simulink model "CalebsModel_v3"  (Simulink 8.3)
settings: Solver=ode45  StartTime=0.0  StopTime=60  RelTol=1e-3
values from neighbouring files (symbols this model uses):
  a_lim = 0.75*F_max/Mar    (= 600)    [ControlDesign.m]
  b_surf = 1e5    (= 100000)    [ControlDesign.m]
  bp = 100    [ControlDesign.m]
  ContactPoint = 0.023    [ControlDesign.m]
  F_max = 60    [ControlDesign.m]
  Home = 0    [ControlDesign.m]
  k_1 = (z_1*z_2-1+k_2*Ts)/(k_2*Ts^2)    [ControlDesign.m]
  k_2 = (2-(z_1+z_2))/Ts    [ControlDesign.m]
  K_backemf = 1000*mean( K_backemf_array )    [ControlDesign.m]
  K_L12_Force = 0.00229181    [ControlDesign.m]    (also in ControlDesignForceModeLinear.m = 2.29181)
  K_PWM = PWM_res/V_rail    (= 83.3333333333)    [ControlDesign.m]    (also in ControlDesignForceModeLinear.m = 0.012)
  k_surf = 1e8    (= 100000000)    [ControlDesign.m]
  kvc = 20e3    (= 20000)    [ControlDesign.m]
  L12_Offset_I = 0.012995    [ControlDesign.m]    (also in ControlDesignForceModeLinear.m = 12.995)
  L_Range = [0 0.050]    [ControlDesign.m]    (also in ControlDesignForceModeLinear.m = [0 50]; VariableQpts.m = [0 50])
  m_surf = 1e3    (= 1000)    [ControlDesign.m]
  Mar = 0.075    [ControlDesign.m]    (also in ControlDesignForceModeLinear.m)
  PWM_res = 2000    [ControlDesign.m]    (also in ControlDesignForceModeLinear.m)
  Ra_L12 = 60    [ControlDesign.m]    (also in ControlDesignForceModeLinear.m)
  Ts = 1/fs    (= 0.001)    [ControlDesign.m]    (also in ControlDesignForceModeLinear.m)
  v_lim = 0.003    [ControlDesign.m]
  ymod = 0.75e-3    (= 0.00075)    [ControlDesign.m]
undefined symbols (not defined in the file or in its folder): DiscIntNeverNeededParam
libraries: simulink x10
settings Model: Creator=secrest  LastModifiedBy=secrest
settings SolverCC: AlgebraicLoopSolver=LineSearch
settings DataIOCC: SignalLoggingSaveFormat=Dataset
settings DebuggingCC: UnderspecifiedInitializationDetection=Simplified  FcnCallInpInsideContextMsg=UseLocalSettings  StateNameClashWarn=none

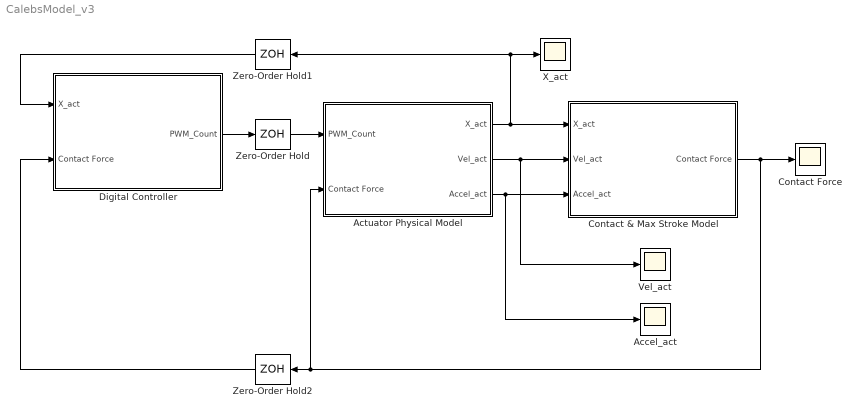
== system CalebsModel_v3 ==
  Accel_act : Scope
      settings: YMin=-100  YMax=1300  SaveName=ScopeData3
  Actuator Physical Model : Subsystem
  Contact & Max Stroke Model : Subsystem
  Contact Force : Scope
      settings: YMin=0  YMax=45
  Digital Controller : Subsystem
  Vel_act : Scope
      settings: YMin=-2.5e-06  YMax=4.25e-05  SaveName=ScopeData2
  X_act : Scope
      settings: YMin=0  YMax=0.017
  Zero-Order Hold : ZeroOrderHold  SampleTime=Ts
  Zero-Order Hold1 : ZeroOrderHold  SampleTime=Ts
  Zero-Order Hold2 : ZeroOrderHold  SampleTime=Ts
  wires:
  Actuator Physical Model/1(X_act) -> Contact & Max Stroke Model/1(X_act), X_act/1, Zero-Order Hold1/1
  Actuator Physical Model/2(Vel_act) -> Contact & Max Stroke Model/2(Vel_act), Vel_act/1
  Actuator Physical Model/3(Accel_act) -> Contact & Max Stroke Model/3(Accel_act), Accel_act/1
  Contact & Max Stroke Model/1(Contact Force) -> Contact Force/1, Actuator Physical Model/2(Contact Force), Zero-Order Hold2/1
  Digital Controller/1(PWM_Count) -> Zero-Order Hold/1
  Zero-Order Hold/1 -> Actuator Physical Model/1(PWM_Count)
  Zero-Order Hold1/1 -> Digital Controller/1(X_act)
  Zero-Order Hold2/1 -> Digital Controller/2(Contact Force)

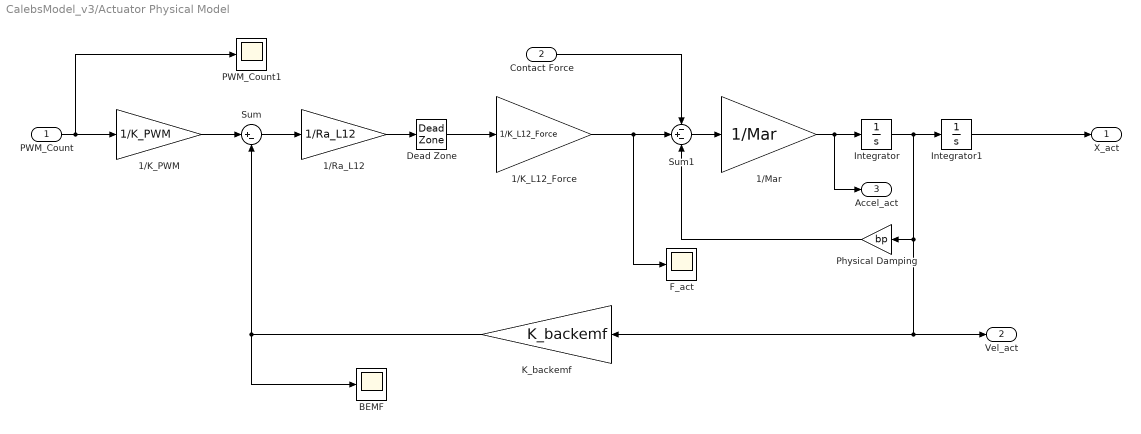
== system CalebsModel_v3/Actuator Physical Model ==
  PWM_Count : Inport
  Contact Force : Inport  Port=2
  1/K_L12_Force : Gain  Gain=1/K_L12_Force
  1/K_PWM : Gain  Gain=1/K_PWM
  1/Mar : Gain  Gain=1/Mar
  1/Ra_L12 : Gain  Gain=1/Ra_L12
  BEMF : Scope
      settings: YMin=0  YMax=100  SaveName=ScopeData8
  Dead Zone : DeadZone  LowerValue=-L12_Offset_I  UpperValue=L12_Offset_I  SaturateOnIntegerOverflow=on
  F_act : Scope
      settings: YMin=0  SaveName=ScopeData5
  Integrator : Integrator
  Integrator1 : Integrator
  K_backemf : Gain  Gain=K_backemf
  PWM_Count1 : Scope
      settings: YMin=-200  YMax=700  SaveName=ScopeData7
  Physical Damping : Gain  Gain=bp
  Sum : Sum  Inputs=|+-
  Sum1 : Sum  Inputs=-+-
  X_act : Outport
  Vel_act : Outport  Port=2
  Accel_act : Outport  Port=3
  wires:
  Sum1/1 -> 1/Mar/1
  1/Ra_L12/1 -> Dead Zone/1
  1/K_PWM/1 -> Sum/1
  Dead Zone/1 -> 1/K_L12_Force/1
  Sum/1 -> 1/Ra_L12/1
  K_backemf/1 -> Sum/2, BEMF/1
  1/K_L12_Force/1 -> F_act/1, Sum1/2
  Integrator1/1 -> X_act/1
  Integrator/1 -> Integrator1/1, Physical Damping/1, K_backemf/1, Vel_act/1
  Contact Force/1 -> Sum1/1
  1/Mar/1 -> Accel_act/1, Integrator/1
  PWM_Count/1 -> PWM_Count1/1, 1/K_PWM/1
  Physical Damping/1 -> Sum1/3

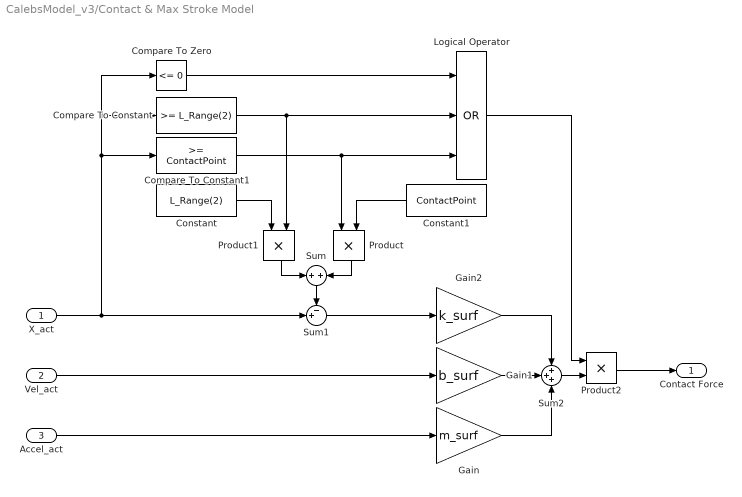
== system CalebsModel_v3/Contact & Max Stroke Model ==
  X_act : Inport
  Vel_act : Inport  Port=2
  Accel_act : Inport  Port=3
  Compare To Constant : simulink/Logic and Bit Operations/Compare To Constant  relop=>=  const=L_Range(2)  OutDataTypeStr=uint8
  Compare To Constant1 : simulink/Logic and Bit Operations/Compare To Constant  relop=>=  const=ContactPoint  OutDataTypeStr=uint8
  Compare To Zero : simulink/Logic and Bit Operations/Compare To Zero  relop=<=  OutDataTypeStr=uint8
  Constant : Constant  Value=L_Range(2)
  Constant1 : Constant  Value=ContactPoint
  Gain : Gain  Gain=m_surf
  Gain1 : Gain  Gain=b_surf
  Gain2 : Gain  Gain=k_surf
  Logical Operator : Logic  Operator=OR  Inputs=3  AllPortsSameDT=off  OutDataTypeStr=boolean
  Product : Product  RndMeth=Zero
  Product1 : Product  RndMeth=Zero
  Product2 : Product  RndMeth=Zero
  Sum : Sum  Inputs=+|+
  Sum1 : Sum  Inputs=-+|
  Sum2 : Sum  Inputs=+++
  Contact Force : Outport
  wires:
  X_act/1 -> Sum1/2, Compare To Zero/1, Compare To Constant/1, Compare To Constant1/1
  Compare To Zero/1 -> Logical Operator/1
  Vel_act/1 -> Gain1/1
  Accel_act/1 -> Gain/1
  Sum/1 -> Sum1/1
  Sum1/1 -> Gain2/1
  Constant/1 -> Product1/1
  Constant1/1 -> Product/2
  Gain2/1 -> Sum2/1
  Gain1/1 -> Sum2/2
  Gain/1 -> Sum2/3
  Logical Operator/1 -> Product2/1
  Sum2/1 -> Product2/2
  Product2/1 -> Contact Force/1
  Compare To Constant/1 -> Logical Operator/2, Product1/2
  Product1/1 -> Sum/1
  Compare To Constant1/1 -> Logical Operator/3, Product/1
  Product/1 -> Sum/2

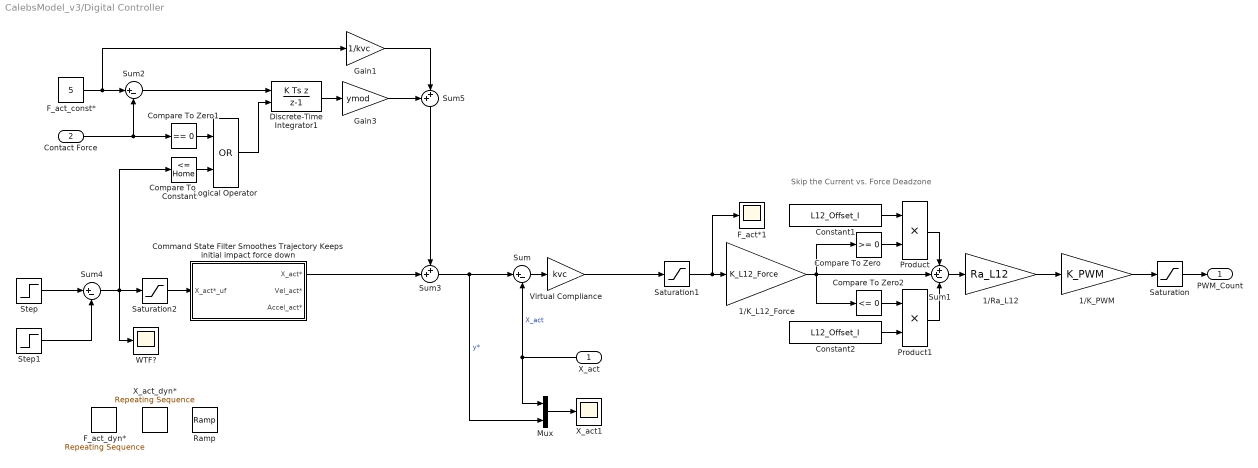
== system CalebsModel_v3/Digital Controller ==
  note: Skip the Current vs. Force Deadzone
  X_act : Inport
  Contact Force : Inport  Port=2
  1/K_L12_Force : Gain  Gain=K_L12_Force
  1/K_PWM : Gain  Gain=K_PWM
  1/Ra_L12 : Gain  Gain=Ra_L12
  Command State Filter Smoothes Trajectory Keeps initial impact force down : Subsystem
  Compare To Constant : simulink/Logic and Bit Operations/Compare To Constant  relop=<=  const=Home  OutDataTypeStr=boolean
  Compare To Zero : simulink/Logic and Bit Operations/Compare To Zero  relop=>=  OutDataTypeStr=uint8
  Compare To Zero1 : simulink/Logic and Bit Operations/Compare To Zero  relop===  OutDataTypeStr=boolean
  Compare To Zero2 : simulink/Logic and Bit Operations/Compare To Zero  relop=<=  OutDataTypeStr=uint8
  Constant1 : Constant  Value=L12_Offset_I
  Constant2 : Constant  Value=L12_Offset_I
  Discrete-Time Integrator1 : DiscreteIntegrator  IntegratorMethod=Integration: Backward Euler  ExternalReset=level  SampleTime=Ts  ICPrevOutput=DiscIntNeverNeededParam  ICPrevScaledInput=DiscIntNeverNeededParam
  F_act*1 : Scope
      settings: YMin=0  YMax=15  SaveName=ScopeData6
  F_act_const* : Constant  Value=5
  F_act_dyn* : simulink/Sources/Repeating Sequence  rep_seq_t=[0 10 15 20 30]  rep_seq_y=[0 0 25 0 0]
  Gain1 : Gain  Gain=1/kvc
  Gain3 : Gain  Gain=ymod
  Logical Operator : Logic  Operator=OR  AllPortsSameDT=off  OutDataTypeStr=boolean
  Mux : Mux  Inputs=2
  Product : Product  RndMeth=Zero
  Product1 : Product  RndMeth=Zero
  Ramp : simulink/Sources/Ramp  slope=0.003  start=1  X0=0
  Saturation : Saturate  UpperLimit=PWM_res  LowerLimit=-PWM_res
  Saturation1 : Saturate  UpperLimit=F_max  LowerLimit=-F_max
  Saturation2 : Saturate  UpperLimit=ContactPoint+0.002  LowerLimit=0
  Step : Step  After=L_Range(2)  SampleTime=0
  Step1 : Step  Time=30  After=L_Range(2)-Home  SampleTime=0
  Sum : Sum  Inputs=|+-
  Sum1 : Sum  Inputs=++-
  Sum2 : Sum  Inputs=|+-
  Sum3 : Sum  Inputs=++|
  Sum4 : Sum  Inputs=|+-
  Sum5 : Sum  Inputs=++|
  Virtual Compliance : Gain  Gain=kvc
  WTF? : Scope
      settings: TimeRange=30  YMin=0  YMax=0.015  SaveName=ScopeData9
  X_act1 : Scope
      settings: TimeRange=30  YMin=-8.67362e-19  YMax=0.0275  SaveName=ScopeData4
  X_act_dyn* : simulink/Sources/Repeating Sequence  rep_seq_t=[0 5 20 25 30]  rep_seq_y=[0 0.006 0.006 0 0]
  PWM_Count : Outport
  wires:
  1/K_PWM/1 -> Saturation/1
  1/K_L12_Force/1 -> Compare To Zero2/1, Sum1/2, Compare To Zero/1
  Constant1/1 -> Product/1
  Compare To Zero/1 -> Product/2
  Product/1 -> Sum1/1
  Sum1/1 -> 1/Ra_L12/1
  Saturation/1 -> PWM_Count/1
  Mux/1 -> X_act1/1
  X_act/1 -> Mux/1, Sum/2  "X_act"
  Sum/1 -> Virtual Compliance/1
  Discrete-Time Integrator1/1 -> Gain3/1
  Saturation1/1 -> F_act*1/1, 1/K_L12_Force/1
  1/Ra_L12/1 -> 1/K_PWM/1
  Sum3/1 -> Sum/1, Mux/2  "y*"
  Command State Filter Smoothes Trajectory Keeps initial impact force down/1(X_act*) -> Sum3/2
  Gain3/1 -> Sum5/1
  Sum5/1 -> Sum3/1
  Gain1/1 -> Sum5/2
  Saturation2/1 -> Command State Filter Smoothes Trajectory Keeps initial impact force down/1(X_act*_uf)
  F_act_const*/1 -> Gain1/1, Sum2/1
  Virtual Compliance/1 -> Saturation1/1
  Sum2/1 -> Discrete-Time Integrator1/1
  Step/1 -> Sum4/1
  Sum4/1 -> WTF?/1, Compare To Constant/1, Saturation2/1
  Product1/1 -> Sum1/3
  Compare To Zero2/1 -> Product1/1
  Constant2/1 -> Product1/2
  Contact Force/1 -> Compare To Zero1/1, Sum2/2
  Step1/1 -> Sum4/2
  Compare To Zero1/1 -> Logical Operator/1
  Compare To Constant/1 -> Logical Operator/2
  Logical Operator/1 -> Discrete-Time Integrator1/2

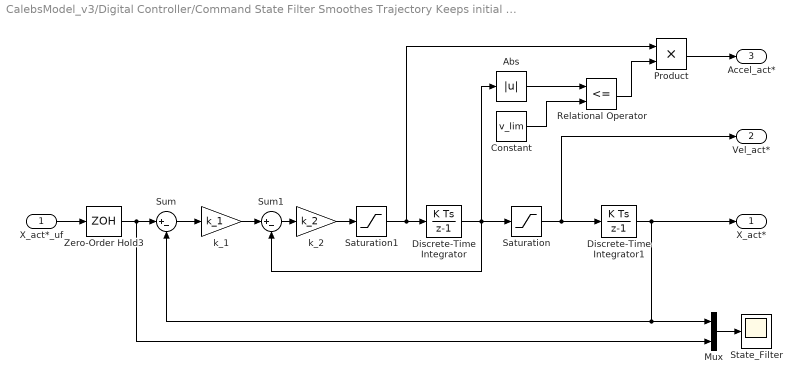
== system CalebsModel_v3/Digital Controller/Command State Filter Smoothes Trajectory Keeps initial impact force down ==
  X_act*_uf : Inport
  Abs : Abs
  Constant : Constant  Value=v_lim
  Discrete-Time Integrator : DiscreteIntegrator  SampleTime=-1  ICPrevOutput=DiscIntNeverNeededParam  ICPrevScaledInput=DiscIntNeverNeededParam
  Discrete-Time Integrator1 : DiscreteIntegrator  SampleTime=-1  ICPrevOutput=DiscIntNeverNeededParam  ICPrevScaledInput=DiscIntNeverNeededParam
  Mux : Mux  Inputs=2
  Product : Product  RndMeth=Zero
  Relational Operator : RelationalOperator  Operator=<=  OutDataTypeStr=boolean
  Saturation : Saturate  UpperLimit=v_lim  LowerLimit=-v_lim
  Saturation1 : Saturate  UpperLimit=a_lim  LowerLimit=-a_lim
  State_Filter : Scope
      settings: YMin=0  YMax=0.006  SaveName=ScopeData2
  Sum : Sum  Inputs=|+-
  Sum1 : Sum  Inputs=|+-
  Zero-Order Hold3 : ZeroOrderHold  SampleTime=Ts
  k_1 : Gain  Gain=k_1
  k_2 : Gain  Gain=k_2
  X_act* : Outport
  Vel_act* : Outport  Port=2
  Accel_act* : Outport  Port=3
  wires:
  Sum/1 -> k_1/1
  k_1/1 -> Sum1/1
  Sum1/1 -> k_2/1
  k_2/1 -> Saturation1/1
  Discrete-Time Integrator/1 -> Sum1/2, Saturation/1, Abs/1
  Discrete-Time Integrator1/1 -> X_act*/1, Sum/2, Mux/1
  Abs/1 -> Relational Operator/1
  Constant/1 -> Relational Operator/2
  Product/1 -> Accel_act*/1
  Saturation/1 -> Discrete-Time Integrator1/1, Vel_act*/1
  Saturation1/1 -> Discrete-Time Integrator/1, Product/1
  Mux/1 -> State_Filter/1
  Zero-Order Hold3/1 -> Sum/1, Mux/2
  X_act*_uf/1 -> Zero-Order Hold3/1
  Relational Operator/1 -> Product/2
